simulink model "XXStIsPos"  (R2018b)
settings: Solver=FixedStepDiscrete  StartTime=0.0  StopTime=10.0  FixedStep=0.01  RelTol=1e-3
settings Model: Creator=sn2xws  LastModifiedBy=sn2xws
settings Model: ModifiedHistory=|
  | V2.1.0
  | Bug541473 增加目标位置为4095时，代表到位置的逻辑
  | V2.5.0
  | 目标位置为4095时，不应该看valid信号
settings DataIOCC: SaveFormat=StructureWithTime
settings OptimizationCC: DefaultParameterBehavior=Inlined  EnhancedBackFolding=on  PassReuseOutputArgsAs=Individual arguments  ZeroExternalMemoryAtStartup=off  ZeroInternalMemoryAtStartup=off  OptimizeBlockOrder=speed  DifferentSizesBufferReuse=on  OptimizationCustomize=off
settings DebuggingCC: ParameterTunabilityLossMsg=error
settings SFSimCC: MATLABDynamicMemAlloc=off
settings RTWCC: SystemTargetFile=autosar.tlc  GenCodeOnly=on  TemplateMakefile=ert_default_tmf  Description=AUTOSAR  GenerateReport=on  IncludeHyperlinkInReport=on  LaunchReport=on  GenerateTraceInfo=on  GenerateTraceReport=on  GenerateTraceReportSl=on  GenerateTraceReportSf=on  GenerateTraceReportEml=on  GenerateCodeMetricsReport=on
settings CodeAppCC: ForceParamTrailComments=on  IgnoreCustomStorageClasses=off  OperatorAnnotations=on  SimulinkDataObjDesc=on  SFDataObjDesc=on  InsertBlockDesc=on
settings STFCustomTargetCC: TargetLangStandard=C99 (ISO)  MultiwordLength=256  ParMdlRefBuildCompliant=on  CompOptLevelCompliant=on  IncludeMdlTerminateFcn=off  CombineOutputUpdateFcns=on  SuppressErrorStatus=on  ERTCustomFileBanners=on  SupportNonFinite=off  SupportComplex=off  SupportContinuousTime=off  SupportNonInlinedSFcns=off  RemoveResetFunc=on  MATLABClassNameForMDSCustomization=Simulink.SoftwareTarget.ERTCustomization  AutosarCompliant=on  UseToolchainInfoCompliant=on  LookupTableObjectStructAxisOrder=2,1,3,4,...  LUTObjectStructOrderEvenSpacing=Size,Table,Breakpoints  SystemTargetFile=autosar.tlc
settings ERTTargetCC: TargetLangStandard=C99 (ISO)  ConcurrentExecutionCompliant=off  IncludeMdlTerminateFcn=off  SuppressErrorStatus=on  SupportNonFinite=off  SupportComplex=off  ModelStepFunctionPrototypeControlCompliant=off  CPPClassGenCompliant=off  AutosarCompliant=on  LookupTableObjectStructAxisOrder=2,1,3,4,...  LUTObjectStructOrderEvenSpacing=Size,Table,Breakpoints  InlinedParameterPlacement=NonHierarchical  ERTCustomFileTemplate=example_file_process.tlc  ERTFilePackagingFormat=Compact

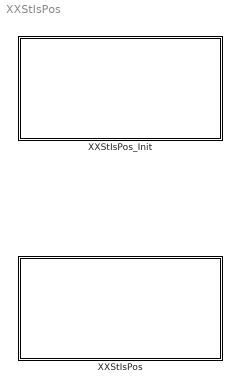
== system XXStIsPos ==
  XXStIsPos : Subsystem
  XXStIsPos_Init : Subsystem

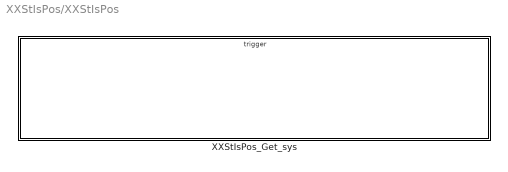
== system XXStIsPos/XXStIsPos ==
  XXStIsPos_Get_sys : Subsystem

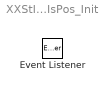
== system XXStIsPos/XXStIsPos_Init ==
  Event Listener : EventListener  EventName=reset

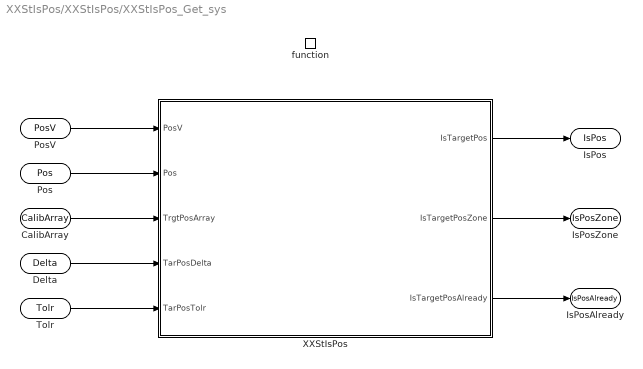
== system XXStIsPos/XXStIsPos/XXStIsPos_Get_sys ==
  function : TriggerPort  TriggerType=function-call  IsSimulinkFunction=on  FunctionName=XXStIsPos_Get  VariantControl=(inherit)
  XXStIsPos : Subsystem
  PosV : ArgIn  OutDataTypeStr=boolean  ArgumentName=PosV
  Pos : ArgIn  Port=2  OutDataTypeStr=uint16  ArgumentName=Pos
  CalibArray : ArgIn  Port=3  OutDataTypeStr=uint16  PortDimensions=3  ArgumentName=CalibArray
  Delta : ArgIn  Port=4  OutDataTypeStr=uint16  ArgumentName=Delta
  Tolr : ArgIn  Port=5  OutDataTypeStr=uint16  ArgumentName=Tolr
  IsPos : ArgOut  OutDataTypeStr=boolean  ArgumentName=IsPos
  IsPosZone : ArgOut  Port=2  OutDataTypeStr=boolean  ArgumentName=IsPosZone
  IsPosAlready : ArgOut  Port=3  OutDataTypeStr=boolean  ArgumentName=IsPosAlready
  wires:
  PosV/1 -> XXStIsPos/1(PosV)
  Pos/1 -> XXStIsPos/2(Pos)
  CalibArray/1 -> XXStIsPos/3(TrgtPosArray)
  Delta/1 -> XXStIsPos/4(TarPosDelta)
  Tolr/1 -> XXStIsPos/5(TarPosTolr)
  XXStIsPos/1(IsTargetPos) -> IsPos/1
  XXStIsPos/3(IsTargetPosAlready) -> IsPosAlready/1
  XXStIsPos/2(IsTargetPosZone) -> IsPosZone/1

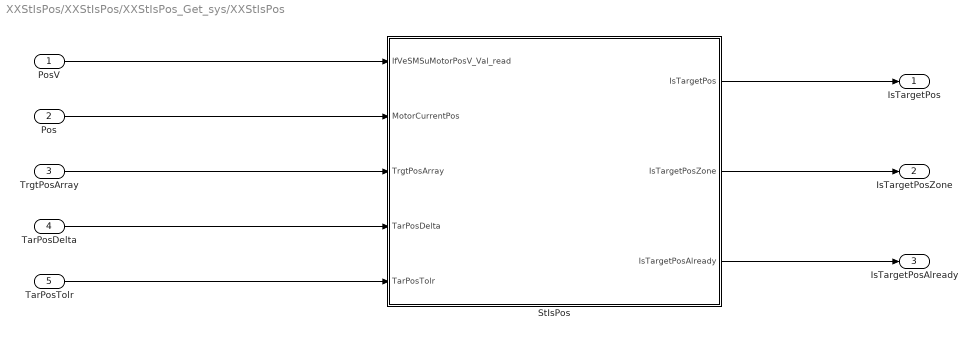
== system XXStIsPos/XXStIsPos/XXStIsPos_Get_sys/XXStIsPos ==
  PosV : Inport
  Pos : Inport  Port=2
  TrgtPosArray : Inport  Port=3
  TarPosDelta : Inport  Port=4
  TarPosTolr : Inport  Port=5
  StIsPos : Subsystem
  IsTargetPos : Outport
  IsTargetPosZone : Outport  Port=2
  IsTargetPosAlready : Outport  Port=3
  wires:
  TarPosTolr/1 -> StIsPos/5(TarPosTolr)
  TrgtPosArray/1 -> StIsPos/3(TrgtPosArray)
  PosV/1 -> StIsPos/1(IfVeSMSuMotorPosV_Val_read)
  TarPosDelta/1 -> StIsPos/4(TarPosDelta)
  Pos/1 -> StIsPos/2(MotorCurrentPos)
  StIsPos/1(IsTargetPos) -> IsTargetPos/1
  StIsPos/3(IsTargetPosAlready) -> IsTargetPosAlready/1
  StIsPos/2(IsTargetPosZone) -> IsTargetPosZone/1

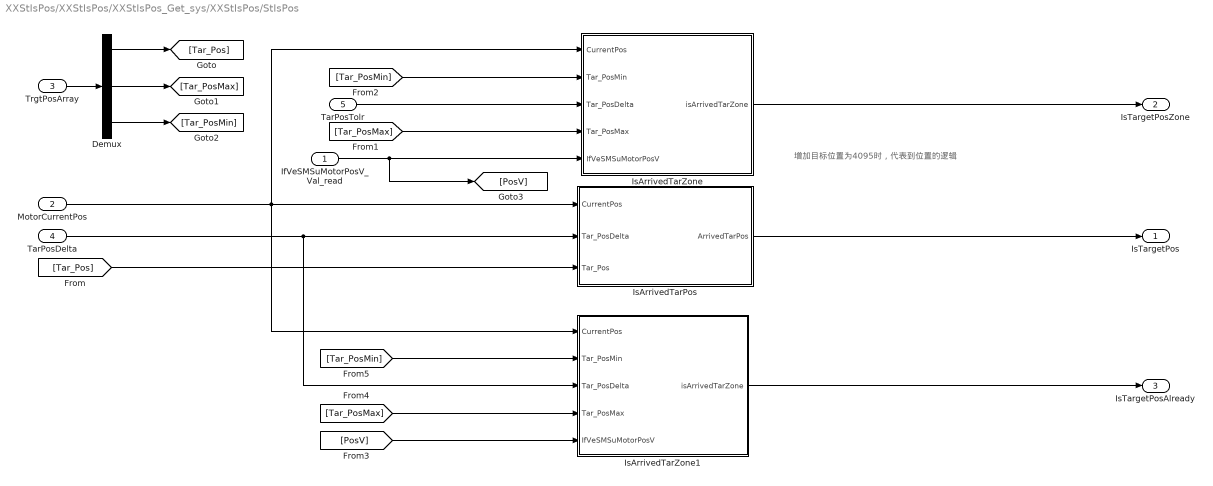
== system XXStIsPos/XXStIsPos/XXStIsPos_Get_sys/XXStIsPos/StIsPos ==
  note: 增加目标位置为4095时，代表到位置的逻辑
  IfVeSMSuMotorPosV_Val_read : Inport
  MotorCurrentPos : Inport  Port=2
  TrgtPosArray : Inport  Port=3
  TarPosDelta : Inport  Port=4
  TarPosTolr : Inport  Port=5
  Demux : Demux  Outputs=3
  IsArrivedTarPos : Subsystem
  IsArrivedTarZone : Subsystem
  IsArrivedTarZone1 : Subsystem
  IsTargetPos : Outport
      settings: EnsureOutportIsVirtual=on
  IsTargetPosZone : Outport  Port=2
      settings: EnsureOutportIsVirtual=on
  IsTargetPosAlready : Outport  Port=3
      settings: EnsureOutportIsVirtual=on
  wires:
  IsArrivedTarZone1/1(isArrivedTarZone) -> IsTargetPosAlready/1
  TarPosTolr/1 -> IsArrivedTarZone/3(Tar_PosDelta)
  TarPosDelta/1 -> IsArrivedTarZone1/3(Tar_PosDelta), IsArrivedTarPos/2(Tar_PosDelta)
  [Tar_PosMin] -> IsArrivedTarZone1/2(Tar_PosMin)
  [Tar_PosMax] -> IsArrivedTarZone1/4(Tar_PosMax)
  [Tar_PosMin] -> IsArrivedTarZone/2(Tar_PosMin)
  [Tar_PosMax] -> IsArrivedTarZone/4(Tar_PosMax)
  [Tar_Pos] -> IsArrivedTarPos/3(Tar_Pos)
  Demux/3 -> [Tar_PosMin]
  Demux/2 -> [Tar_PosMax]
  Demux/1 -> [Tar_Pos]
  TrgtPosArray/1 -> Demux/1
  IsArrivedTarZone/1(isArrivedTarZone) -> IsTargetPosZone/1
  IsArrivedTarPos/1(ArrivedTarPos) -> IsTargetPos/1
  MotorCurrentPos/1 -> IsArrivedTarZone1/1(CurrentPos), IsArrivedTarPos/1(CurrentPos), IsArrivedTarZone/1(CurrentPos)
  IfVeSMSuMotorPosV_Val_read/1 -> [PosV], IsArrivedTarZone/5(IfVeSMSuMotorPosV)
  [PosV] -> IsArrivedTarZone1/5(IfVeSMSuMotorPosV)

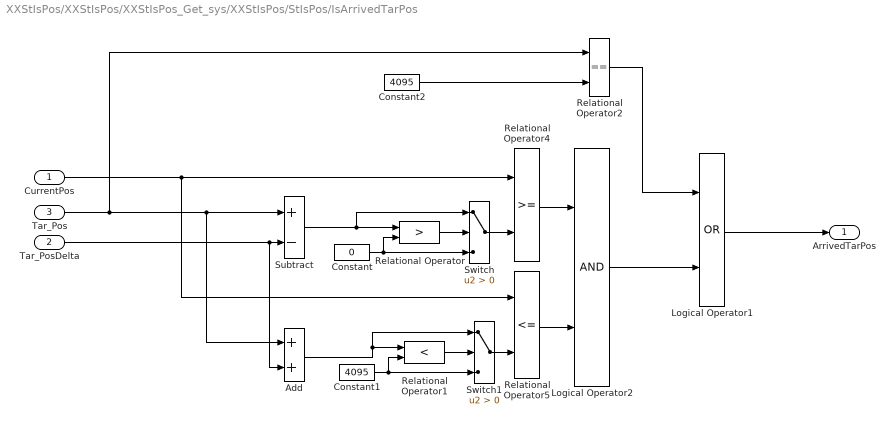
== system XXStIsPos/XXStIsPos/XXStIsPos_Get_sys/XXStIsPos/StIsPos/IsArrivedTarPos ==
  CurrentPos : Inport
  Tar_PosDelta : Inport  Port=2
  Tar_Pos : Inport  Port=3
  Add : Sum
  Constant : Constant  Value=0  OutDataTypeStr=uint16
  Constant1 : Constant  Value=4095  OutDataTypeStr=uint16
  Constant2 : Constant  Value=4095  OutDataTypeStr=uint16
  Logical Operator1 : Logic  Operator=OR  AllPortsSameDT=off  OutDataTypeStr=boolean
  Logical Operator2 : Logic  AllPortsSameDT=off  OutDataTypeStr=boolean
  Relational Operator : RelationalOperator  Operator=>  OutDataTypeStr=boolean  RndMeth=Simplest
  Relational Operator1 : RelationalOperator  Operator=<  OutDataTypeStr=boolean  RndMeth=Simplest
  Relational Operator2 : RelationalOperator  Operator===  OutDataTypeStr=boolean  RndMeth=Simplest
  Relational Operator4 : RelationalOperator  OutDataTypeStr=boolean  RndMeth=Simplest
  Relational Operator5 : RelationalOperator  Operator=<=  OutDataTypeStr=boolean  RndMeth=Simplest
  Subtract : Sum  Inputs=+-  OutDataTypeStr=int16
  Switch : Switch  Criteria=u2 > Threshold
  Switch1 : Switch  Criteria=u2 > Threshold
  ArrivedTarPos : Outport
  wires:
  Relational Operator1/1 -> Switch1/2
  Switch1/1 -> Relational Operator5/2
  Constant1/1 -> Switch1/3, Relational Operator1/2
  Add/1 -> Relational Operator1/1, Switch1/1
  Constant/1 -> Switch/3, Relational Operator/2
  Relational Operator/1 -> Switch/2
  Subtract/1 -> Relational Operator/1, Switch/1
  CurrentPos/1 -> Relational Operator5/1, Relational Operator4/1
  Switch/1 -> Relational Operator4/2
  Tar_PosDelta/1 -> Subtract/2, Add/2
  Relational Operator4/1 -> Logical Operator2/1
  Relational Operator5/1 -> Logical Operator2/2
  Tar_Pos/1 -> Relational Operator2/1, Subtract/1, Add/1
  Constant2/1 -> Relational Operator2/2
  Logical Operator1/1 -> ArrivedTarPos/1
  Logical Operator2/1 -> Logical Operator1/2
  Relational Operator2/1 -> Logical Operator1/1

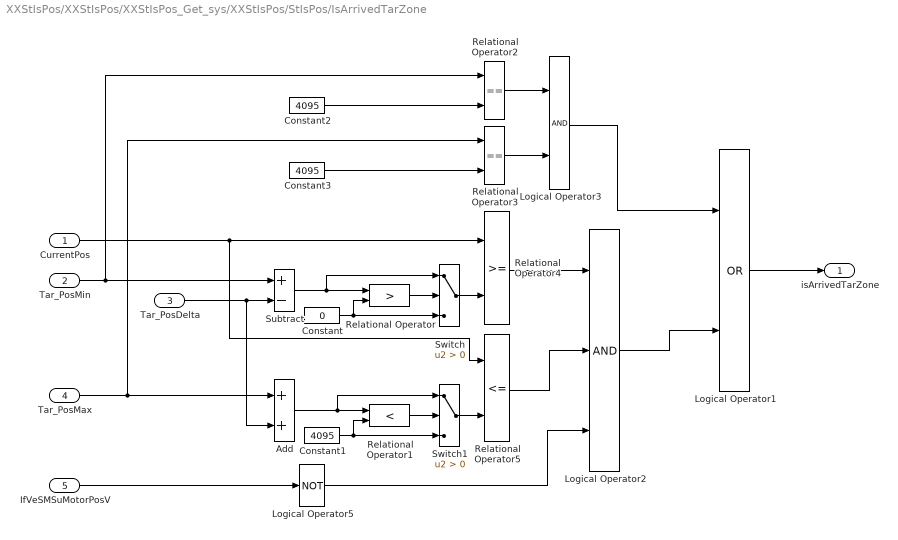
== system XXStIsPos/XXStIsPos/XXStIsPos_Get_sys/XXStIsPos/StIsPos/IsArrivedTarZone ==
  CurrentPos : Inport
  Tar_PosMin : Inport  Port=2
  Tar_PosDelta : Inport  Port=3
  Tar_PosMax : Inport  Port=4
  IfVeSMSuMotorPosV : Inport  Port=5
  Add : Sum
  Constant : Constant  Value=0  OutDataTypeStr=uint16
  Constant1 : Constant  Value=4095  OutDataTypeStr=uint16
  Constant2 : Constant  Value=4095  OutDataTypeStr=uint16
  Constant3 : Constant  Value=4095  OutDataTypeStr=uint16
  Logical Operator1 : Logic  Operator=OR  AllPortsSameDT=off  OutDataTypeStr=boolean
  Logical Operator2 : Logic  Inputs=3  AllPortsSameDT=off  OutDataTypeStr=boolean
  Logical Operator3 : Logic  AllPortsSameDT=off  OutDataTypeStr=boolean
  Logical Operator5 : Logic  Operator=NOT  AllPortsSameDT=off  OutDataTypeStr=boolean
  Relational Operator : RelationalOperator  Operator=>  OutDataTypeStr=boolean  RndMeth=Simplest
  Relational Operator1 : RelationalOperator  Operator=<  OutDataTypeStr=boolean  RndMeth=Simplest
  Relational Operator2 : RelationalOperator  Operator===  OutDataTypeStr=boolean  RndMeth=Simplest
  Relational Operator3 : RelationalOperator  Operator===  OutDataTypeStr=boolean  RndMeth=Simplest
  Relational Operator4 : RelationalOperator  OutDataTypeStr=boolean  RndMeth=Simplest
  Relational Operator5 : RelationalOperator  Operator=<=  OutDataTypeStr=boolean  RndMeth=Simplest
  Subtract : Sum  Inputs=+-  OutDataTypeStr=int16
  Switch : Switch  Criteria=u2 > Threshold
  Switch1 : Switch  Criteria=u2 > Threshold
  isArrivedTarZone : Outport
  wires:
  Constant1/1 -> Switch1/3, Relational Operator1/2
  Relational Operator1/1 -> Switch1/2
  Relational Operator/1 -> Switch/2
  Constant/1 -> Switch/3, Relational Operator/2
  Subtract/1 -> Relational Operator/1, Switch/1
  Relational Operator4/1 -> Logical Operator2/1
  Tar_PosMax/1 -> Relational Operator3/1, Add/1
  Relational Operator5/1 -> Logical Operator2/2
  Switch/1 -> Relational Operator4/2
  Tar_PosMin/1 -> Relational Operator2/1, Subtract/1
  CurrentPos/1 -> Relational Operator5/1, Relational Operator4/1
  Switch1/1 -> Relational Operator5/2
  Add/1 -> Relational Operator1/1, Switch1/1
  Tar_PosDelta/1 -> Add/2, Subtract/2
  Logical Operator1/1 -> isArrivedTarZone/1
  Constant2/1 -> Relational Operator2/2
  Constant3/1 -> Relational Operator3/2
  Relational Operator2/1 -> Logical Operator3/1
  Relational Operator3/1 -> Logical Operator3/2
  Logical Operator3/1 -> Logical Operator1/1
  IfVeSMSuMotorPosV/1 -> Logical Operator5/1
  Logical Operator5/1 -> Logical Operator2/3
  Logical Operator2/1 -> Logical Operator1/2

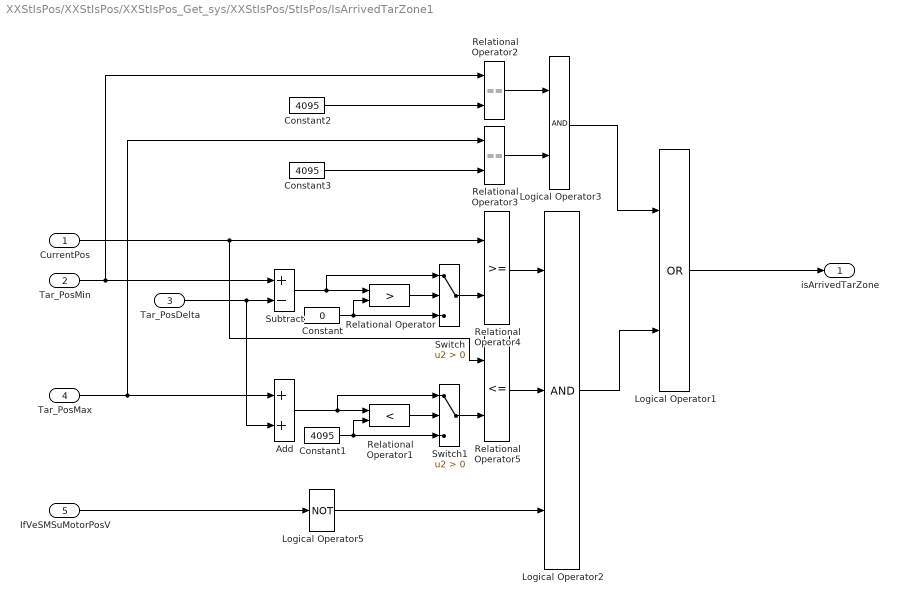
== system XXStIsPos/XXStIsPos/XXStIsPos_Get_sys/XXStIsPos/StIsPos/IsArrivedTarZone1 ==
  CurrentPos : Inport
  Tar_PosMin : Inport  Port=2
  Tar_PosDelta : Inport  Port=3
  Tar_PosMax : Inport  Port=4
  IfVeSMSuMotorPosV : Inport  Port=5
  Add : Sum
  Constant : Constant  Value=0  OutDataTypeStr=uint16
  Constant1 : Constant  Value=4095  OutDataTypeStr=uint16
  Constant2 : Constant  Value=4095  OutDataTypeStr=uint16
  Constant3 : Constant  Value=4095  OutDataTypeStr=uint16
  Logical Operator1 : Logic  Operator=OR  AllPortsSameDT=off  OutDataTypeStr=boolean
  Logical Operator2 : Logic  Inputs=3  AllPortsSameDT=off  OutDataTypeStr=boolean
  Logical Operator3 : Logic  AllPortsSameDT=off  OutDataTypeStr=boolean
  Logical Operator5 : Logic  Operator=NOT  AllPortsSameDT=off  OutDataTypeStr=boolean
  Relational Operator : RelationalOperator  Operator=>  OutDataTypeStr=boolean  RndMeth=Simplest
  Relational Operator1 : RelationalOperator  Operator=<  OutDataTypeStr=boolean  RndMeth=Simplest
  Relational Operator2 : RelationalOperator  Operator===  OutDataTypeStr=boolean  RndMeth=Simplest
  Relational Operator3 : RelationalOperator  Operator===  OutDataTypeStr=boolean  RndMeth=Simplest
  Relational Operator4 : RelationalOperator  OutDataTypeStr=boolean  RndMeth=Simplest
  Relational Operator5 : RelationalOperator  Operator=<=  OutDataTypeStr=boolean  RndMeth=Simplest
  Subtract : Sum  Inputs=+-  OutDataTypeStr=int16
  Switch : Switch  Criteria=u2 > Threshold
  Switch1 : Switch  Criteria=u2 > Threshold
  isArrivedTarZone : Outport
  wires:
  Logical Operator3/1 -> Logical Operator1/1
  Relational Operator3/1 -> Logical Operator3/2
  Relational Operator2/1 -> Logical Operator3/1
  Constant3/1 -> Relational Operator3/2
  Constant2/1 -> Relational Operator2/2
  Logical Operator2/1 -> Logical Operator1/2
  Logical Operator1/1 -> isArrivedTarZone/1
  Tar_PosDelta/1 -> Subtract/2, Add/2
  Add/1 -> Switch1/1, Relational Operator1/1
  Switch1/1 -> Relational Operator5/2
  CurrentPos/1 -> Relational Operator4/1, Relational Operator5/1
  Tar_PosMin/1 -> Subtract/1, Relational Operator2/1
  Switch/1 -> Relational Operator4/2
  Relational Operator5/1 -> Logical Operator2/2
  Tar_PosMax/1 -> Add/1, Relational Operator3/1
  Relational Operator4/1 -> Logical Operator2/1
  Subtract/1 -> Switch/1, Relational Operator/1
  Constant/1 -> Relational Operator/2, Switch/3
  Relational Operator/1 -> Switch/2
  Relational Operator1/1 -> Switch1/2
  Constant1/1 -> Relational Operator1/2, Switch1/3
  IfVeSMSuMotorPosV/1 -> Logical Operator5/1
  Logical Operator5/1 -> Logical Operator2/3
